simulink model "quadplane_sim_conf"  (R2023a)
settings: Solver=FixedStepAuto  StartTime=0.0  StopTime=100  FixedStep=0.001  RelTol=1e-9
undefined symbols (not defined in the file or in its folder): Aircraft, datetime, datevec, Earth, Env, Fmu, framePeriod_s, InitCond, Telem, WGS84
libraries: simulink x9, aerolibconvert2 x5, aerolibasang x3, aerolibtransform2 x2, aerolibatmos2 x1, aerolibgravity2 x1, sharedtransform x1, uavutilslib x1, aerolibadyn x1, fuzblock x1, shared6dof x1
(part 3 of 5)

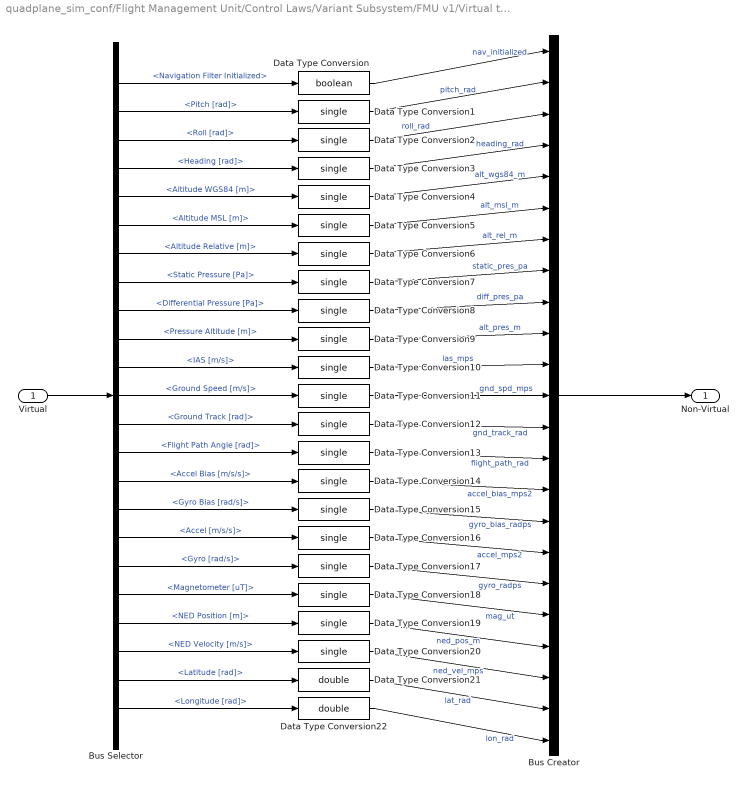
== system quadplane_sim_conf/Flight Management Unit/Control Laws/Variant Subsystem/FMU v1/Virtual to Non-Virtual Mapping2 ==
  Virtual : Inport
  Bus Creator : BusCreator  Inputs=23  OutDataTypeStr=Bus: NavData  NonVirtualBus=on
  Bus Selector : BusSelector  OutputSignals=Navigation Filter Initialized,Pitch [rad],Roll [rad],Heading [rad],Altitude WGS84 [m],Altitude MSL [m],Altitude Relative [m],Static Pressure [Pa],Differential Pressure [Pa],Pressure Altitude [m],IAS [m/s],Ground Speed [m/s],Ground Track [rad],Flight Path Angle [rad],Accel Bias [m/s/s],Gyro Bias [rad/s],Accel [m/s/s],Gyro [rad/s],Magnetometer [uT],NED Position [m],NED Velocity [m/s],Latitude [rad],Longitude [rad]
  Data Type Conversion : DataTypeConversion  OutDataTypeStr=boolean  SaturateOnIntegerOverflow=off  RndMeth=Floor
  Data Type Conversion{1..20} (20 alike) : DataTypeConversion  OutDataTypeStr=single  SaturateOnIntegerOverflow=off  RndMeth=Floor
  Data Type Conversion21 : DataTypeConversion  OutDataTypeStr=double  SaturateOnIntegerOverflow=off  RndMeth=Floor
  Data Type Conversion22 : DataTypeConversion  OutDataTypeStr=double  SaturateOnIntegerOverflow=off  RndMeth=Floor
  Non-Virtual : Outport  OutDataTypeStr=Bus: NavData
  wires:
  Data Type Conversion17/1 -> Bus Creator/18  "gyro_radps"
  Data Type Conversion22/1 -> Bus Creator/23  "lon_rad"
  Data Type Conversion21/1 -> Bus Creator/22  "lat_rad"
  Data Type Conversion20/1 -> Bus Creator/21  "ned_vel_mps"
  Data Type Conversion19/1 -> Bus Creator/20  "ned_pos_m"
  Data Type Conversion18/1 -> Bus Creator/19  "mag_ut"
  Data Type Conversion16/1 -> Bus Creator/17  "accel_mps2"
  Data Type Conversion15/1 -> Bus Creator/16  "gyro_bias_radps"
  Data Type Conversion14/1 -> Bus Creator/15  "accel_bias_mps2"
  Data Type Conversion13/1 -> Bus Creator/14  "flight_path_rad"
  Data Type Conversion12/1 -> Bus Creator/13  "gnd_track_rad"
  Data Type Conversion11/1 -> Bus Creator/12  "gnd_spd_mps"
  Data Type Conversion10/1 -> Bus Creator/11  "ias_mps"
  Data Type Conversion9/1 -> Bus Creator/10  "alt_pres_m"
  Data Type Conversion8/1 -> Bus Creator/9  "diff_pres_pa"
  Data Type Conversion7/1 -> Bus Creator/8  "static_pres_pa"
  Data Type Conversion6/1 -> Bus Creator/7  "alt_rel_m"
  Data Type Conversion5/1 -> Bus Creator/6  "alt_msl_m"
  Data Type Conversion4/1 -> Bus Creator/5  "alt_wgs84_m"
  Data Type Conversion3/1 -> Bus Creator/4  "heading_rad"
  Data Type Conversion2/1 -> Bus Creator/3  "roll_rad"
  Data Type Conversion1/1 -> Bus Creator/2  "pitch_rad"
  Data Type Conversion/1 -> Bus Creator/1  "nav_initialized"
  Bus Selector/23 -> Data Type Conversion22/1  "<Longitude [rad]>"
  Bus Selector/22 -> Data Type Conversion21/1  "<Latitude [rad]>"
  Bus Selector/21 -> Data Type Conversion20/1  "<NED Velocity [m/s]>"
  Bus Selector/20 -> Data Type Conversion19/1  "<NED Position [m]>"
  Bus Selector/19 -> Data Type Conversion18/1  "<Magnetometer [uT]>"
  Bus Selector/18 -> Data Type Conversion17/1  "<Gyro [rad/s]>"
  Bus Selector/17 -> Data Type Conversion16/1  "<Accel [m/s/s]>"
  Bus Selector/16 -> Data Type Conversion15/1  "<Gyro Bias [rad/s]>"
  Bus Selector/15 -> Data Type Conversion14/1  "<Accel Bias [m/s/s]>"
  Bus Selector/14 -> Data Type Conversion13/1  "<Flight Path Angle [rad]>"
  Bus Selector/13 -> Data Type Conversion12/1  "<Ground Track [rad]>"
  Bus Selector/12 -> Data Type Conversion11/1  "<Ground Speed [m/s]>"
  Bus Selector/11 -> Data Type Conversion10/1  "<IAS [m/s]>"
  Bus Selector/10 -> Data Type Conversion9/1  "<Pressure Altitude [m]>"
  Bus Selector/9 -> Data Type Conversion8/1  "<Differential Pressure [Pa]>"
  Bus Selector/8 -> Data Type Conversion7/1  "<Static Pressure [Pa]>"
  Bus Selector/7 -> Data Type Conversion6/1  "<Altitude Relative [m]>"
  Bus Selector/6 -> Data Type Conversion5/1  "<Altitude MSL [m]>"
  Bus Selector/5 -> Data Type Conversion4/1  "<Altitude WGS84 [m]>"
  Bus Selector/4 -> Data Type Conversion3/1  "<Heading [rad]>"
  Bus Selector/3 -> Data Type Conversion2/1  "<Roll [rad]>"
  Bus Selector/2 -> Data Type Conversion1/1  "<Pitch [rad]>"
  Bus Selector/1 -> Data Type Conversion/1  "<Navigation Filter Initialized>"
  Bus Creator/1 -> Non-Virtual/1
  Virtual/1 -> Bus Selector/1

== system quadplane_sim_conf/Flight Management Unit/Control Laws/Variant Subsystem/FMU v1/Virtual to Non-Virtual Mapping3 ==
  Virtual : Inport
  Bus Creator : BusCreator  Inputs=11  OutDataTypeStr=Bus: TelemData  NonVirtualBus=on
  Bus Selector : BusSelector  OutputSignals=Waypoints Updated,Fence Updated,Rally Points Updated,Current Waypoint Index,Number of Waypoints,Number of Fence Points,Number of Rally Points,Parameters,Flight Plan,Fence,Rally
  Data Type Conversion : DataTypeConversion  OutDataTypeStr=boolean  SaturateOnIntegerOverflow=off  RndMeth=Floor
  Data Type Conversion1 : DataTypeConversion  OutDataTypeStr=boolean  SaturateOnIntegerOverflow=off  RndMeth=Floor
  Data Type Conversion2 : DataTypeConversion  OutDataTypeStr=boolean  SaturateOnIntegerOverflow=off  RndMeth=Floor
  Data Type Conversion{3..6} (4 alike) : DataTypeConversion  OutDataTypeStr=int16  SaturateOnIntegerOverflow=off  RndMeth=Floor
  Data Type Conversion7 : DataTypeConversion  OutDataTypeStr=single  SaturateOnIntegerOverflow=off  RndMeth=Floor
  Signal Conversion : SignalConversion  ConversionOutput=Nonvirtual bus  OverrideOpt=off
  Signal Conversion1 : SignalConversion  ConversionOutput=Nonvirtual bus  OverrideOpt=off
  Signal Conversion2 : SignalConversion  ConversionOutput=Nonvirtual bus  OverrideOpt=off
  Non-Virtual : Outport  OutDataTypeStr=Bus: TelemData
  wires:
  Signal Conversion2/1 -> Bus Creator/11  "rally"
  Signal Conversion1/1 -> Bus Creator/10  "fence"
  Signal Conversion/1 -> Bus Creator/9  "flight_plan"
  Bus Selector/11 -> Signal Conversion2/1  "<Rally>"
  Bus Selector/10 -> Signal Conversion1/1  "<Fence>"
  Bus Selector/9 -> Signal Conversion/1  "<Flight Plan>"
  Data Type Conversion7/1 -> Bus Creator/8  "param"
  Data Type Conversion6/1 -> Bus Creator/7  "num_rally_points"
  Data Type Conversion5/1 -> Bus Creator/6  "num_fence_items"
  Data Type Conversion4/1 -> Bus Creator/5  "num_waypoints"
  Data Type Conversion3/1 -> Bus Creator/4  "current_waypoint"
  Data Type Conversion2/1 -> Bus Creator/3  "rally_points_updated"
  Data Type Conversion1/1 -> Bus Creator/2  "fence_updated"
  Data Type Conversion/1 -> Bus Creator/1  "waypoints_updated"
  Bus Selector/8 -> Data Type Conversion7/1  "<Parameters>"
  Bus Selector/7 -> Data Type Conversion6/1  "<Number of Rally Points>"
  Bus Selector/6 -> Data Type Conversion5/1  "<Number of Fence Points>"
  Bus Selector/5 -> Data Type Conversion4/1  "<Number of Waypoints>"
  Bus Selector/4 -> Data Type Conversion3/1  "<Current Waypoint Index>"
  Bus Selector/3 -> Data Type Conversion2/1  "<Rally Points Updated>"
  Bus Selector/2 -> Data Type Conversion1/1  "<Fence Updated>"
  Bus Selector/1 -> Data Type Conversion/1  "<Waypoints Updated>"
  Bus Creator/1 -> Non-Virtual/1
  Virtual/1 -> Bus Selector/1

== system quadplane_sim_conf/Flight Management Unit/Control Laws/Variant Subsystem/FMU v1/Virtual to Non-Virtual Mapping4 ==
  Non-Virtual : Inport  OutDataTypeStr=Bus: ControlData
  Bus Creator : BusCreator  Inputs=5
  Bus Selector : BusSelector  OutputSignals=waypoint_reached,mode,sbus,pwm,aux
  Data Type Conversion{1..4,22} (5 alike) : DataTypeConversion  OutDataTypeStr=double  SaturateOnIntegerOverflow=off  RndMeth=Floor
  Virtual : Outport
  wires:
  Data Type Conversion4/1 -> Bus Creator/5  "AUX"
  Data Type Conversion3/1 -> Bus Creator/4  "PWM"
  Bus Selector/5 -> Data Type Conversion4/1  "<aux>"
  Bus Selector/4 -> Data Type Conversion3/1  "<pwm>"
  Data Type Conversion2/1 -> Bus Creator/3  "SBUS"
  Bus Selector/3 -> Data Type Conversion2/1  "<sbus>"
  Data Type Conversion1/1 -> Bus Creator/2  "Mode"
  Bus Selector/2 -> Data Type Conversion1/1  "<mode>"
  Data Type Conversion22/1 -> Bus Creator/1  "Waypoint Reached"
  Bus Selector/1 -> Data Type Conversion22/1  "<waypoint_reached>"
  Bus Creator/1 -> Virtual/1
  Non-Virtual/1 -> Bus Selector/1

== system quadplane_sim_conf/Flight Management Unit/Control Laws/Variant Subsystem/FMU v1/Virtual to Non-Virtual Mapping5 ==
  Virtual : Inport
  Bus Creator : BusCreator  Inputs=7  OutDataTypeStr=Bus: SensorData  NonVirtualBus=on
  Bus Selector : BusSelector  OutputSignals=Pitot Static Installed,Inceptor,IMU,GNSS,Static Pressure,Differential Pressure,Analog
  Data Type Conversion : DataTypeConversion  OutDataTypeStr=boolean  SaturateOnIntegerOverflow=off  RndMeth=Floor
  Virtual to Non-Virtual Mapping1 : Subsystem
  Virtual to Non-Virtual Mapping2 : Subsystem
  Virtual to Non-Virtual Mapping3 : Subsystem
  Virtual to Non-Virtual Mapping4 : Subsystem
  Virtual to Non-Virtual Mapping5 : Subsystem
  Virtual to Non-Virtual Mapping6 : Subsystem
  Non-Virtual : Outport  OutDataTypeStr=Bus: SensorData
  wires:
  Virtual/1 -> Bus Selector/1
  Bus Creator/1 -> Non-Virtual/1
  Bus Selector/1 -> Data Type Conversion/1  "<Pitot Static Installed>"
  Data Type Conversion/1 -> Bus Creator/1  "pitot_static_installed"
  Bus Selector/2 -> Virtual to Non-Virtual Mapping1/1(Virtual)  "<Inceptor>"
  Virtual to Non-Virtual Mapping1/1(Non-Virtual) -> Bus Creator/2  "inceptor"
  Virtual to Non-Virtual Mapping2/1(Non-Virtual) -> Bus Creator/3  "imu"
  Bus Selector/3 -> Virtual to Non-Virtual Mapping2/1(Virtual)  "<IMU>"
  Virtual to Non-Virtual Mapping3/1(Non-Virtual) -> Bus Creator/4  "gnss"
  Bus Selector/4 -> Virtual to Non-Virtual Mapping3/1(Virtual)  "<GNSS>"
  Virtual to Non-Virtual Mapping4/1(Non-Virtual) -> Bus Creator/5  "static_pres"
  Bus Selector/5 -> Virtual to Non-Virtual Mapping4/1(Virtual)  "<Static Pressure>"
  Virtual to Non-Virtual Mapping5/1(Non-Virtual) -> Bus Creator/6  "diff_pres"
  Bus Selector/6 -> Virtual to Non-Virtual Mapping5/1(Virtual)  "<Differential Pressure>"
  Bus Selector/7 -> Virtual to Non-Virtual Mapping6/1(Virtual)  "<Analog>"
  Virtual to Non-Virtual Mapping6/1(Non-Virtual) -> Bus Creator/7  "adc"

== system quadplane_sim_conf/Flight Management Unit/Control Laws/Variant Subsystem/FMU v2/Virtual to Non-Virtual Mapping ==
  Virtual : Inport
  Bus Creator : BusCreator  Inputs=2  OutDataTypeStr=Bus: SysData  NonVirtualBus=on
  Bus Selector : BusSelector  OutputSignals=Frame Time [us],System Time [us]
  Data Type Conversion : DataTypeConversion  OutDataTypeStr=int32  SaturateOnIntegerOverflow=off  RndMeth=Floor
  Data Type Conversion5 : DataTypeConversion  OutDataTypeStr=int64  SaturateOnIntegerOverflow=off  RndMeth=Floor
  Non-Virtual : Outport  OutDataTypeStr=Bus: SysData
  wires:
  Bus Creator/1 -> Non-Virtual/1
  Virtual/1 -> Bus Selector/1
  Bus Selector/1 -> Data Type Conversion/1  "<Frame Time [us]>"
  Data Type Conversion/1 -> Bus Creator/1  "frame_time_us"
  Bus Selector/2 -> Data Type Conversion5/1  "<System Time [us]>"
  Data Type Conversion5/1 -> Bus Creator/2  "sys_time_us"

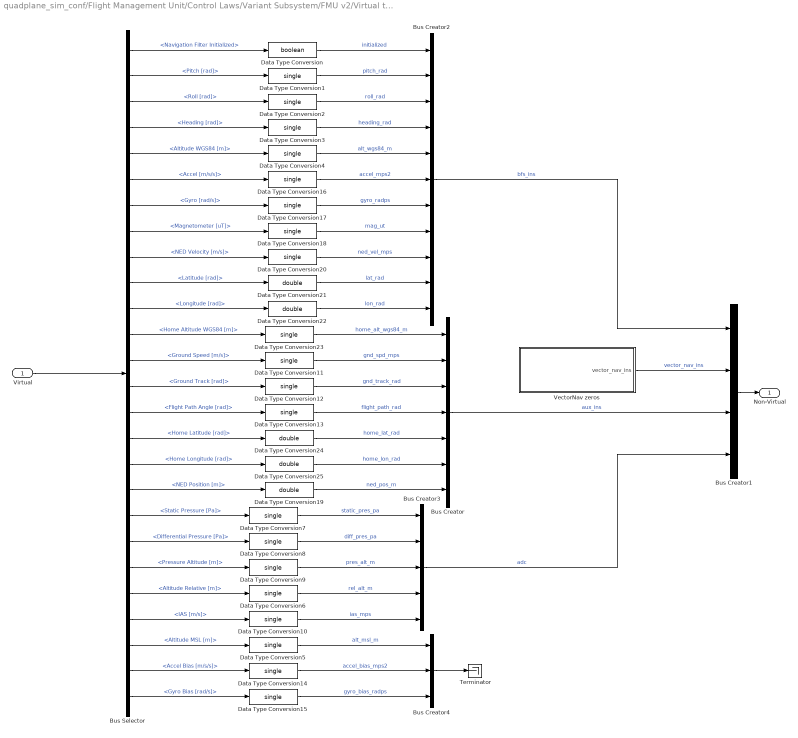
== system quadplane_sim_conf/Flight Management Unit/Control Laws/Variant Subsystem/FMU v2/Virtual to Non-Virtual Mapping1 ==
  Virtual : Inport
  Bus Creator : BusCreator  Inputs=7  OutDataTypeStr=Bus: AuxInsData
  Bus Creator1 : BusCreator  Inputs=4  OutDataTypeStr=Bus: StateEstData
  Bus Creator2 : BusCreator  Inputs=11  OutDataTypeStr=Bus: InsData
  Bus Creator3 : BusCreator  Inputs=5  OutDataTypeStr=Bus: AdcData
  Bus Creator4 : BusCreator  Inputs=3
  Bus Selector : BusSelector  OutputSignals=Navigation Filter Initialized,Pitch [rad],Roll [rad],Heading [rad],Altitude WGS84 [m],Accel [m/s/s],Gyro [rad/s],Magnetometer [uT],NED Velocity [m/s],Latitude [rad],Longitude [rad],Home Altitude WGS84 [m],Ground Speed [m/s],Ground Track [rad],Flight Path Angle [rad],Home Latitude [rad],Home Longitude [rad],NED Position [m],Static Pressure [Pa],Differential Pressure [Pa],Pressure Altitude [m],Altitude Relative [m],IAS [m/s],Altitude MSL [m],Accel Bias [m/s/s],Gyro Bias [rad/s]
  Data Type Conversion : DataTypeConversion  OutDataTypeStr=boolean  SaturateOnIntegerOverflow=off  RndMeth=Floor
  Data Type Conversion{1..18,20,23} (20 alike) : DataTypeConversion  OutDataTypeStr=single  SaturateOnIntegerOverflow=off  RndMeth=Floor
  Data Type Conversion{19,21..22,24..25} (5 alike) : DataTypeConversion  OutDataTypeStr=double  SaturateOnIntegerOverflow=off  RndMeth=Floor
  Terminator : Terminator
  VectorNav zeros : Subsystem
  Non-Virtual : Outport  OutDataTypeStr=Bus: StateEstData
  wires:
  Virtual/1 -> Bus Selector/1
  Bus Selector/1 -> Data Type Conversion/1  "<Navigation Filter Initialized>"
  Bus Selector/2 -> Data Type Conversion1/1  "<Pitch [rad]>"
  Bus Selector/3 -> Data Type Conversion2/1  "<Roll [rad]>"
  Bus Selector/4 -> Data Type Conversion3/1  "<Heading [rad]>"
  Bus Selector/5 -> Data Type Conversion4/1  "<Altitude WGS84 [m]>"
  Bus Selector/24 -> Data Type Conversion5/1  "<Altitude MSL [m]>"
  Bus Selector/22 -> Data Type Conversion6/1  "<Altitude Relative [m]>"
  Bus Selector/19 -> Data Type Conversion7/1  "<Static Pressure [Pa]>"
  Bus Selector/20 -> Data Type Conversion8/1  "<Differential Pressure [Pa]>"
  Bus Selector/21 -> Data Type Conversion9/1  "<Pressure Altitude [m]>"
  Bus Selector/23 -> Data Type Conversion10/1  "<IAS [m/s]>"
  Bus Selector/13 -> Data Type Conversion11/1  "<Ground Speed [m/s]>"
  Bus Selector/14 -> Data Type Conversion12/1  "<Ground Track [rad]>"
  Bus Selector/15 -> Data Type Conversion13/1  "<Flight Path Angle [rad]>"
  Bus Selector/25 -> Data Type Conversion14/1  "<Accel Bias [m/s/s]>"
  Bus Selector/26 -> Data Type Conversion15/1  "<Gyro Bias [rad/s]>"
  Bus Selector/6 -> Data Type Conversion16/1  "<Accel [m/s/s]>"
  Bus Selector/7 -> Data Type Conversion17/1  "<Gyro [rad/s]>"
  Bus Selector/8 -> Data Type Conversion18/1  "<Magnetometer [uT]>"
  Bus Selector/18 -> Data Type Conversion19/1  "<NED Position [m]>"
  Bus Selector/9 -> Data Type Conversion20/1  "<NED Velocity [m/s]>"
  Bus Selector/10 -> Data Type Conversion21/1  "<Latitude [rad]>"
  Bus Selector/11 -> Data Type Conversion22/1  "<Longitude [rad]>"
  Data Type Conversion/1 -> Bus Creator2/1  "initialized"
  Data Type Conversion1/1 -> Bus Creator2/2  "pitch_rad"
  Data Type Conversion2/1 -> Bus Creator2/3  "roll_rad"
  Data Type Conversion3/1 -> Bus Creator2/4  "heading_rad"
  Data Type Conversion4/1 -> Bus Creator2/5  "alt_wgs84_m"
  Data Type Conversion22/1 -> Bus Creator2/11  "lon_rad"
  Data Type Conversion21/1 -> Bus Creator2/10  "lat_rad"
  Data Type Conversion20/1 -> Bus Creator2/9  "ned_vel_mps"
  Data Type Conversion19/1 -> Bus Creator/7  "ned_pos_m"
  Data Type Conversion18/1 -> Bus Creator2/8  "mag_ut"
  Data Type Conversion17/1 -> Bus Creator2/7  "gyro_radps"
  Data Type Conversion16/1 -> Bus Creator2/6  "accel_mps2"
  Data Type Conversion15/1 -> Bus Creator4/3  "gyro_bias_radps"
  Data Type Conversion14/1 -> Bus Creator4/2  "accel_bias_mps2"
  Data Type Conversion13/1 -> Bus Creator/4  "flight_path_rad"
  Data Type Conversion12/1 -> Bus Creator/3  "gnd_track_rad"
  Data Type Conversion11/1 -> Bus Creator/2  "gnd_spd_mps"
  Data Type Conversion10/1 -> Bus Creator3/5  "ias_mps"
  Data Type Conversion9/1 -> Bus Creator3/3  "pres_alt_m"
  Data Type Conversion8/1 -> Bus Creator3/2  "diff_pres_pa"
  Data Type Conversion7/1 -> Bus Creator3/1  "static_pres_pa"
  Data Type Conversion6/1 -> Bus Creator3/4  "rel_alt_m"
  Bus Selector/12 -> Data Type Conversion23/1  "<Home Altitude WGS84 [m]>"
  Data Type Conversion23/1 -> Bus Creator/1  "home_alt_wgs84_m"
  Bus Selector/16 -> Data Type Conversion24/1  "<Home Latitude [rad]>"
  Bus Selector/17 -> Data Type Conversion25/1  "<Home Longitude [rad]>"
  Data Type Conversion24/1 -> Bus Creator/5  "home_lat_rad"
  Data Type Conversion25/1 -> Bus Creator/6  "home_lon_rad"
  Bus Creator1/1 -> Non-Virtual/1
  Bus Creator2/1 -> Bus Creator1/1  "bfs_ins"
  Data Type Conversion5/1 -> Bus Creator4/1  "alt_msl_m"
  Bus Creator/1 -> Bus Creator1/3  "aux_ins"
  Bus Creator3/1 -> Bus Creator1/4  "adc"
  Bus Creator4/1 -> Terminator/1
  VectorNav zeros/1(vector_nav_ins) -> Bus Creator1/2  "vector_nav_ins"

== system quadplane_sim_conf/Flight Management Unit/Control Laws/Variant Subsystem/FMU v2/Virtual to Non-Virtual Mapping3 ==
  Virtual : Inport
  Bus Creator : BusCreator  Inputs=11  OutDataTypeStr=Bus: TelemData  NonVirtualBus=on
  Bus Selector : BusSelector  OutputSignals=Waypoints Updated,Fence Updated,Rally Points Updated,Current Waypoint Index,Number of Waypoints,Number of Fence Points,Number of Rally Points,Parameters,Flight Plan,Fence,Rally
  Data Type Conversion : DataTypeConversion  OutDataTypeStr=boolean  SaturateOnIntegerOverflow=off  RndMeth=Floor
  Data Type Conversion1 : DataTypeConversion  OutDataTypeStr=boolean  SaturateOnIntegerOverflow=off  RndMeth=Floor
  Data Type Conversion2 : DataTypeConversion  OutDataTypeStr=boolean  SaturateOnIntegerOverflow=off  RndMeth=Floor
  Data Type Conversion{3..6} (4 alike) : DataTypeConversion  OutDataTypeStr=int16  SaturateOnIntegerOverflow=off  RndMeth=Floor
  Data Type Conversion7 : DataTypeConversion  OutDataTypeStr=single  SaturateOnIntegerOverflow=off  RndMeth=Floor
  Signal Conversion : SignalConversion  ConversionOutput=Nonvirtual bus  OutDataTypeStr=Bus: MissionItem  OverrideOpt=off
  Signal Conversion1 : SignalConversion  ConversionOutput=Nonvirtual bus  OutDataTypeStr=Bus: MissionItem  OverrideOpt=off
  Signal Conversion2 : SignalConversion  ConversionOutput=Nonvirtual bus  OutDataTypeStr=Bus: MissionItem  OverrideOpt=off
  Non-Virtual : Outport  OutDataTypeStr=Bus: TelemData
  wires:
  Virtual/1 -> Bus Selector/1
  Bus Creator/1 -> Non-Virtual/1
  Bus Selector/1 -> Data Type Conversion/1  "<Waypoints Updated>"
  Bus Selector/2 -> Data Type Conversion1/1  "<Fence Updated>"
  Bus Selector/3 -> Data Type Conversion2/1  "<Rally Points Updated>"
  Bus Selector/4 -> Data Type Conversion3/1  "<Current Waypoint Index>"
  Bus Selector/5 -> Data Type Conversion4/1  "<Number of Waypoints>"
  Bus Selector/6 -> Data Type Conversion5/1  "<Number of Fence Points>"
  Bus Selector/7 -> Data Type Conversion6/1  "<Number of Rally Points>"
  Bus Selector/8 -> Data Type Conversion7/1  "<Parameters>"
  Data Type Conversion/1 -> Bus Creator/1  "waypoints_updated"
  Data Type Conversion1/1 -> Bus Creator/2  "fence_updated"
  Data Type Conversion2/1 -> Bus Creator/3  "rally_points_updated"
  Data Type Conversion3/1 -> Bus Creator/4  "current_waypoint"
  Data Type Conversion4/1 -> Bus Creator/5  "num_waypoints"
  Data Type Conversion5/1 -> Bus Creator/6  "num_fence_items"
  Data Type Conversion6/1 -> Bus Creator/7  "num_rally_points"
  Data Type Conversion7/1 -> Bus Creator/8  "param"
  Bus Selector/9 -> Signal Conversion/1  "<Flight Plan>"
  Bus Selector/10 -> Signal Conversion1/1  "<Fence>"
  Bus Selector/11 -> Signal Conversion2/1  "<Rally>"
  Signal Conversion/1 -> Bus Creator/9  "flight_plan"
  Signal Conversion1/1 -> Bus Creator/10  "fence"
  Signal Conversion2/1 -> Bus Creator/11  "rally"

== system quadplane_sim_conf/Flight Management Unit/Control Laws/Variant Subsystem/FMU v2/Virtual to Non-Virtual Mapping4 ==
  Non-Virtual1 : Inport  OutDataTypeStr=Bus: VmsData
  Bus Creator1 : BusCreator  Inputs=9
  Bus Selector1 : BusSelector  OutputSignals=advance_waypoint,motors_enabled,mode,sbus,pwm,throttle_cmd_prcnt,flight_time_remaining_s,power_remaining_prcnt,aux
  Cast To Boolean : DataTypeConversion  OutDataTypeStr=boolean  SaturateOnIntegerOverflow=off  RndMeth=Floor
  Cast To Boolean1 : DataTypeConversion  OutDataTypeStr=boolean  SaturateOnIntegerOverflow=off  RndMeth=Floor
  Cast To Boolean2 : DataTypeConversion  OutDataTypeStr=int8  SaturateOnIntegerOverflow=off  RndMeth=Floor
  Cast To Boolean3 : DataTypeConversion  OutDataTypeStr=int16  SaturateOnIntegerOverflow=off  RndMeth=Floor
  Cast To Boolean4 : DataTypeConversion  OutDataTypeStr=int16  SaturateOnIntegerOverflow=off  RndMeth=Floor
  Cast To Boolean{5..8} (4 alike) : DataTypeConversion  OutDataTypeStr=single  SaturateOnIntegerOverflow=off  RndMeth=Floor
  Virtual1 : Outport
  wires:
  Non-Virtual1/1 -> Bus Selector1/1
  Bus Creator1/1 -> Virtual1/1
  Bus Selector1/1 -> Cast To Boolean/1  "<advance_waypoint>"
  Bus Selector1/2 -> Cast To Boolean1/1  "<motors_enabled>"
  Bus Selector1/3 -> Cast To Boolean2/1  "<mode>"
  Bus Selector1/4 -> Cast To Boolean3/1  "<sbus>"
  Bus Selector1/5 -> Cast To Boolean4/1  "<pwm>"
  Bus Selector1/6 -> Cast To Boolean5/1  "<throttle_cmd_prcnt>"
  Bus Selector1/7 -> Cast To Boolean6/1  "<flight_time_remaining_s>"
  Bus Selector1/8 -> Cast To Boolean7/1  "<power_remaining_prcnt>"
  Bus Selector1/9 -> Cast To Boolean8/1  "<aux>"
  Cast To Boolean/1 -> Bus Creator1/1  "advance_waypoint"
  Cast To Boolean1/1 -> Bus Creator1/2  "motors-enabled"
  Cast To Boolean2/1 -> Bus Creator1/3  "mode"
  Cast To Boolean3/1 -> Bus Creator1/4  "sbus"
  Cast To Boolean4/1 -> Bus Creator1/5  "pwm"
  Cast To Boolean5/1 -> Bus Creator1/6  "throttle_cmd_prcnt"
  Cast To Boolean6/1 -> Bus Creator1/7  "flight_time_remaining_s"
  Cast To Boolean7/1 -> Bus Creator1/8  "power_remaining_prcnt"
  Cast To Boolean8/1 -> Bus Creator1/9  "aux"

== system quadplane_sim_conf/Flight Management Unit/Control Laws/Variant Subsystem/FMU v2/Virtual to Non-Virtual Mapping5 ==
  Virtual : Inport
  Bus Creator : BusCreator  Inputs=18  OutDataTypeStr=Bus: SensorData
  Bus Selector : BusSelector  OutputSignals=Pitot Static Installed,Inceptor,IMU,Static Pressure,GNSS,Differential Pressure,Analog,Battery
  Subsystem : Subsystem
  Subsystem1 : Subsystem
  Subsystem2 : Subsystem
  Subsystem3 : Subsystem
  Subsystem4 : Subsystem
  Subsystem5 : Subsystem
  Subsystem6 : Subsystem
  Subsystem7 : Subsystem
  ZEROS : Subsystem
  Non-Virtual : Outport  OutDataTypeStr=Bus: SensorData
  wires:
  Virtual/1 -> Bus Selector/1
  Bus Creator/1 -> Non-Virtual/1
  Bus Selector/1 -> [pitot_static_installed]  "<Pitot Static Installed>"
  Bus Selector/2 -> Subsystem/1(In1)  "<Inceptor>"
  Subsystem/1(Out1) -> Bus Creator/1
  Bus Selector/7 -> Subsystem1/1(In1)  "<Analog>"
  Bus Selector/3 -> Subsystem6/1(In1), Subsystem5/1(In1)  "<IMU>"
  Bus Selector/5 -> Subsystem7/1(In1)  "<GNSS>"
  Subsystem1/1(Out1) -> Bus Creator/17
  Bus Selector/8 -> Subsystem2/1(<Battery>)  "<Battery>"
  Subsystem2/1(Out1) -> Bus Creator/18
  Bus Selector/4 -> Subsystem3/1(In1)  "<Static Pressure>"
  Bus Selector/6 -> Subsystem4/2(In1)  "<Differential Pressure>"
  Subsystem7/1(Out1) -> Bus Creator/10
  Subsystem4/1(Out1) -> Bus Creator/13
  Subsystem3/1(Out1) -> Bus Creator/4
  Subsystem5/1(Out1) -> Bus Creator/2
  Subsystem6/1(Out1) -> Bus Creator/3
  ZEROS/3(GNSS) -> Bus Creator/11, Bus Creator/8
  ZEROS/4(ExtPres) -> Bus Creator/7, Bus Creator/15, Bus Creator/14, Bus Creator/12
  ZEROS/2(MAG) -> Bus Creator/9, Bus Creator/6
  ZEROS/1(IMU) -> Bus Creator/5
  ZEROS/5(RadAlt) -> Bus Creator/16
  [pitot_static_installed] -> Subsystem4/1(In2)

== system quadplane_sim_conf/Flight Management Unit/Control Laws/Variant Subsystem/FMU v2 Beta/Virtual to Non-Virtual Mapping ==
  Virtual : Inport
  Bus Creator : BusCreator  Inputs=4  OutDataTypeStr=Bus: SysData  NonVirtualBus=on
  Bus Selector : BusSelector  OutputSignals=Frame Time [us],Frame Time [s],System Time [us],System Time [s]
  Data Type Conversion : DataTypeConversion  OutDataTypeStr=int32  SaturateOnIntegerOverflow=off  RndMeth=Floor
  Data Type Conversion5 : DataTypeConversion  OutDataTypeStr=int64  SaturateOnIntegerOverflow=off  RndMeth=Floor
  Data Type Conversion6 : DataTypeConversion  OutDataTypeStr=single  SaturateOnIntegerOverflow=off  RndMeth=Floor
  Data Type Conversion7 : DataTypeConversion  OutDataTypeStr=double  SaturateOnIntegerOverflow=off  RndMeth=Floor
  Non-Virtual : Outport  OutDataTypeStr=Bus: SysData
  wires:
  Bus Creator/1 -> Non-Virtual/1
  Virtual/1 -> Bus Selector/1
  Bus Selector/1 -> Data Type Conversion/1  "<Frame Time [us]>"
  Data Type Conversion/1 -> Bus Creator/1  "frame_time_us"
  Bus Selector/3 -> Data Type Conversion5/1  "<System Time [us]>"
  Data Type Conversion5/1 -> Bus Creator/3  "sys_time_us"
  Bus Selector/2 -> Data Type Conversion6/1  "<Frame Time [s]>"
  Data Type Conversion6/1 -> Bus Creator/2  "frame_time_s"
  Bus Selector/4 -> Data Type Conversion7/1  "<System Time [s]>"
  Data Type Conversion7/1 -> Bus Creator/4  "sys_time_s"

== system quadplane_sim_conf/Flight Management Unit/Control Laws/Variant Subsystem/FMU v2 Beta/Virtual to Non-Virtual Mapping1 ==
  Virtual : Inport
  Bus Creator : BusCreator  Inputs=7  OutDataTypeStr=Bus: SensorData  NonVirtualBus=on
  Bus Selector : BusSelector  OutputSignals=Pitot Static Installed,Inceptor,IMU,GNSS,Static Pressure,Differential Pressure,Analog
  Data Type Conversion : DataTypeConversion  OutDataTypeStr=boolean  SaturateOnIntegerOverflow=off  RndMeth=Floor
  Virtual to Non-Virtual Mapping1 : Subsystem
  Virtual to Non-Virtual Mapping2 : Subsystem
  Virtual to Non-Virtual Mapping3 : Subsystem
  Virtual to Non-Virtual Mapping4 : Subsystem
  Virtual to Non-Virtual Mapping5 : Subsystem
  Virtual to Non-Virtual Mapping6 : Subsystem
  Non-Virtual : Outport  OutDataTypeStr=Bus: SensorData
  wires:
  Virtual/1 -> Bus Selector/1
  Bus Creator/1 -> Non-Virtual/1
  Bus Selector/1 -> Data Type Conversion/1  "<Pitot Static Installed>"
  Data Type Conversion/1 -> Bus Creator/1  "pitot_static_installed"
  Bus Selector/2 -> Virtual to Non-Virtual Mapping1/1(Virtual)  "<Inceptor>"
  Virtual to Non-Virtual Mapping1/1(Non-Virtual) -> Bus Creator/2  "inceptor"
  Virtual to Non-Virtual Mapping2/1(Non-Virtual) -> Bus Creator/3  "imu"
  Bus Selector/3 -> Virtual to Non-Virtual Mapping2/1(Virtual)  "<IMU>"
  Virtual to Non-Virtual Mapping3/1(Non-Virtual) -> Bus Creator/4  "gnss"
  Bus Selector/4 -> Virtual to Non-Virtual Mapping3/1(Virtual)  "<GNSS>"
  Virtual to Non-Virtual Mapping4/1(Non-Virtual) -> Bus Creator/5  "static_pres"
  Bus Selector/5 -> Virtual to Non-Virtual Mapping4/1(Virtual)  "<Static Pressure>"
  Virtual to Non-Virtual Mapping5/1(Non-Virtual) -> Bus Creator/6  "diff_pres"
  Bus Selector/6 -> Virtual to Non-Virtual Mapping5/1(Virtual)  "<Differential Pressure>"
  Bus Selector/7 -> Virtual to Non-Virtual Mapping6/1(Virtual)  "<Analog>"
  Virtual to Non-Virtual Mapping6/1(Non-Virtual) -> Bus Creator/7  "analog"

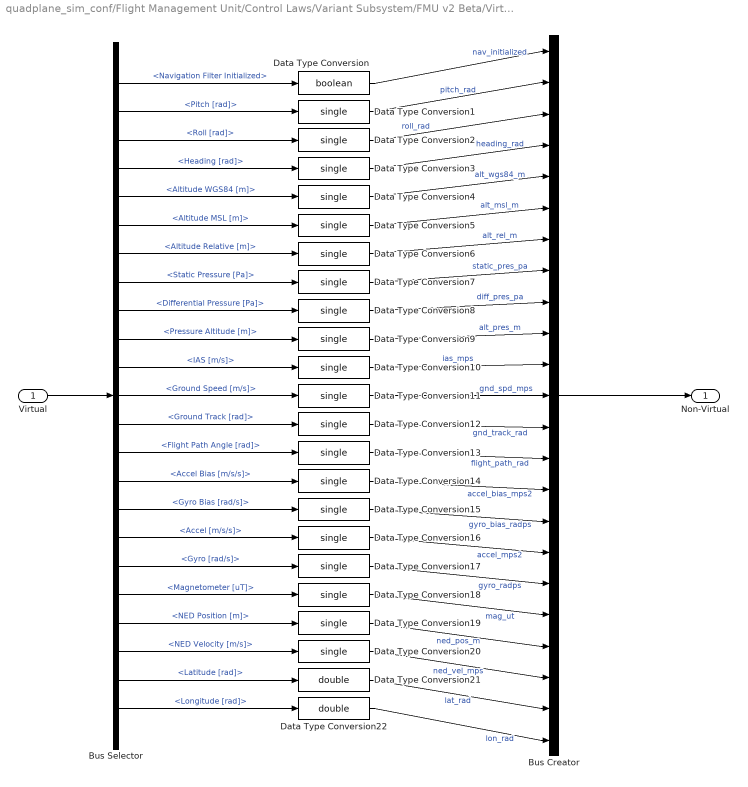
== system quadplane_sim_conf/Flight Management Unit/Control Laws/Variant Subsystem/FMU v2 Beta/Virtual to Non-Virtual Mapping2 ==
  Virtual : Inport
  Bus Creator : BusCreator  Inputs=23  OutDataTypeStr=Bus: NavData  NonVirtualBus=on
  Bus Selector : BusSelector  OutputSignals=Navigation Filter Initialized,Pitch [rad],Roll [rad],Heading [rad],Altitude WGS84 [m],Altitude MSL [m],Altitude Relative [m],Static Pressure [Pa],Differential Pressure [Pa],Pressure Altitude [m],IAS [m/s],Ground Speed [m/s],Ground Track [rad],Flight Path Angle [rad],Accel Bias [m/s/s],Gyro Bias [rad/s],Accel [m/s/s],Gyro [rad/s],Magnetometer [uT],NED Position [m],NED Velocity [m/s],Latitude [rad],Longitude [rad]
  Data Type Conversion : DataTypeConversion  OutDataTypeStr=boolean  SaturateOnIntegerOverflow=off  RndMeth=Floor
  Data Type Conversion{1..20} (20 alike) : DataTypeConversion  OutDataTypeStr=single  SaturateOnIntegerOverflow=off  RndMeth=Floor
  Data Type Conversion21 : DataTypeConversion  OutDataTypeStr=double  SaturateOnIntegerOverflow=off  RndMeth=Floor
  Data Type Conversion22 : DataTypeConversion  OutDataTypeStr=double  SaturateOnIntegerOverflow=off  RndMeth=Floor
  Non-Virtual : Outport  OutDataTypeStr=Bus: NavData
  wires:
  Virtual/1 -> Bus Selector/1
  Bus Creator/1 -> Non-Virtual/1
  Bus Selector/1 -> Data Type Conversion/1  "<Navigation Filter Initialized>"
  Bus Selector/2 -> Data Type Conversion1/1  "<Pitch [rad]>"
  Bus Selector/3 -> Data Type Conversion2/1  "<Roll [rad]>"
  Bus Selector/4 -> Data Type Conversion3/1  "<Heading [rad]>"
  Bus Selector/5 -> Data Type Conversion4/1  "<Altitude WGS84 [m]>"
  Bus Selector/6 -> Data Type Conversion5/1  "<Altitude MSL [m]>"
  Bus Selector/7 -> Data Type Conversion6/1  "<Altitude Relative [m]>"
  Bus Selector/8 -> Data Type Conversion7/1  "<Static Pressure [Pa]>"
  Bus Selector/9 -> Data Type Conversion8/1  "<Differential Pressure [Pa]>"
  Bus Selector/10 -> Data Type Conversion9/1  "<Pressure Altitude [m]>"
  Bus Selector/11 -> Data Type Conversion10/1  "<IAS [m/s]>"
  Bus Selector/12 -> Data Type Conversion11/1  "<Ground Speed [m/s]>"
  Bus Selector/13 -> Data Type Conversion12/1  "<Ground Track [rad]>"
  Bus Selector/14 -> Data Type Conversion13/1  "<Flight Path Angle [rad]>"
  Bus Selector/15 -> Data Type Conversion14/1  "<Accel Bias [m/s/s]>"
  Bus Selector/16 -> Data Type Conversion15/1  "<Gyro Bias [rad/s]>"
  Bus Selector/17 -> Data Type Conversion16/1  "<Accel [m/s/s]>"
  Bus Selector/18 -> Data Type Conversion17/1  "<Gyro [rad/s]>"
  Bus Selector/19 -> Data Type Conversion18/1  "<Magnetometer [uT]>"
  Bus Selector/20 -> Data Type Conversion19/1  "<NED Position [m]>"
  Bus Selector/21 -> Data Type Conversion20/1  "<NED Velocity [m/s]>"
  Bus Selector/22 -> Data Type Conversion21/1  "<Latitude [rad]>"
  Bus Selector/23 -> Data Type Conversion22/1  "<Longitude [rad]>"
  Data Type Conversion/1 -> Bus Creator/1  "nav_initialized"
  Data Type Conversion1/1 -> Bus Creator/2  "pitch_rad"
  Data Type Conversion2/1 -> Bus Creator/3  "roll_rad"
  Data Type Conversion3/1 -> Bus Creator/4  "heading_rad"
  Data Type Conversion4/1 -> Bus Creator/5  "alt_wgs84_m"
  Data Type Conversion5/1 -> Bus Creator/6  "alt_msl_m"
  Data Type Conversion6/1 -> Bus Creator/7  "alt_rel_m"
  Data Type Conversion7/1 -> Bus Creator/8  "static_pres_pa"
  Data Type Conversion8/1 -> Bus Creator/9  "diff_pres_pa"
  Data Type Conversion9/1 -> Bus Creator/10  "alt_pres_m"
  Data Type Conversion10/1 -> Bus Creator/11  "ias_mps"
  Data Type Conversion11/1 -> Bus Creator/12  "gnd_spd_mps"
  Data Type Conversion12/1 -> Bus Creator/13  "gnd_track_rad"
  Data Type Conversion13/1 -> Bus Creator/14  "flight_path_rad"
  Data Type Conversion14/1 -> Bus Creator/15  "accel_bias_mps2"
  Data Type Conversion15/1 -> Bus Creator/16  "gyro_bias_radps"
  Data Type Conversion16/1 -> Bus Creator/17  "accel_mps2"
  Data Type Conversion18/1 -> Bus Creator/19  "mag_ut"
  Data Type Conversion19/1 -> Bus Creator/20  "ned_pos_m"
  Data Type Conversion20/1 -> Bus Creator/21  "ned_vel_mps"
  Data Type Conversion21/1 -> Bus Creator/22  "lat_rad"
  Data Type Conversion22/1 -> Bus Creator/23  "lon_rad"
  Data Type Conversion17/1 -> Bus Creator/18  "gyro_radps"

== system quadplane_sim_conf/Flight Management Unit/Control Laws/Variant Subsystem/FMU v2 Beta/Virtual to Non-Virtual Mapping3 ==
  Virtual : Inport
  Bus Creator : BusCreator  Inputs=11  OutDataTypeStr=Bus: TelemData  NonVirtualBus=on
  Bus Selector : BusSelector  OutputSignals=Waypoints Updated,Fence Updated,Rally Points Updated,Current Waypoint Index,Number of Waypoints,Number of Fence Points,Number of Rally Points,Parameters,Flight Plan,Fence,Rally
  Data Type Conversion : DataTypeConversion  OutDataTypeStr=boolean  SaturateOnIntegerOverflow=off  RndMeth=Floor
  Data Type Conversion1 : DataTypeConversion  OutDataTypeStr=boolean  SaturateOnIntegerOverflow=off  RndMeth=Floor
  Data Type Conversion2 : DataTypeConversion  OutDataTypeStr=boolean  SaturateOnIntegerOverflow=off  RndMeth=Floor
  Data Type Conversion{3..6} (4 alike) : DataTypeConversion  OutDataTypeStr=int16  SaturateOnIntegerOverflow=off  RndMeth=Floor
  Data Type Conversion7 : DataTypeConversion  OutDataTypeStr=single  SaturateOnIntegerOverflow=off  RndMeth=Floor
  Signal Conversion : SignalConversion  ConversionOutput=Nonvirtual bus  OverrideOpt=off
  Signal Conversion1 : SignalConversion  ConversionOutput=Nonvirtual bus  OverrideOpt=off
  Signal Conversion2 : SignalConversion  ConversionOutput=Nonvirtual bus  OverrideOpt=off
  Non-Virtual : Outport  OutDataTypeStr=Bus: TelemData
  wires:
  Virtual/1 -> Bus Selector/1
  Bus Creator/1 -> Non-Virtual/1
  Bus Selector/1 -> Data Type Conversion/1  "<Waypoints Updated>"
  Bus Selector/2 -> Data Type Conversion1/1  "<Fence Updated>"
  Bus Selector/3 -> Data Type Conversion2/1  "<Rally Points Updated>"
  Bus Selector/4 -> Data Type Conversion3/1  "<Current Waypoint Index>"
  Bus Selector/5 -> Data Type Conversion4/1  "<Number of Waypoints>"
  Bus Selector/6 -> Data Type Conversion5/1  "<Number of Fence Points>"
  Bus Selector/7 -> Data Type Conversion6/1  "<Number of Rally Points>"
  Bus Selector/8 -> Data Type Conversion7/1  "<Parameters>"
  Data Type Conversion/1 -> Bus Creator/1  "waypoints_updated"
  Data Type Conversion1/1 -> Bus Creator/2  "fence_updated"
  Data Type Conversion2/1 -> Bus Creator/3  "rally_points_updated"
  Data Type Conversion3/1 -> Bus Creator/4  "current_waypoint"
  Data Type Conversion4/1 -> Bus Creator/5  "num_waypoints"
  Data Type Conversion5/1 -> Bus Creator/6  "num_fence_items"
  Data Type Conversion6/1 -> Bus Creator/7  "num_rally_points"
  Data Type Conversion7/1 -> Bus Creator/8  "param"
  Bus Selector/9 -> Signal Conversion/1  "<Flight Plan>"
  Bus Selector/10 -> Signal Conversion1/1  "<Fence>"
  Bus Selector/11 -> Signal Conversion2/1  "<Rally>"
  Signal Conversion/1 -> Bus Creator/9  "flight_plan"
  Signal Conversion1/1 -> Bus Creator/10  "fence"
  Signal Conversion2/1 -> Bus Creator/11  "rally"

== system quadplane_sim_conf/Flight Management Unit/Control Laws/Variant Subsystem/FMU v2 Beta/Virtual to Non-Virtual Mapping4 ==
  Non-Virtual : Inport  OutDataTypeStr=Bus: ControlData
  Bus Creator : BusCreator  Inputs=5
  Bus Selector : BusSelector  OutputSignals=waypoint_reached,mode,sbus,pwm,aux
  Data Type Conversion{1..4,22} (5 alike) : DataTypeConversion  OutDataTypeStr=double  SaturateOnIntegerOverflow=off  RndMeth=Floor
  Virtual : Outport
  wires:
  Non-Virtual/1 -> Bus Selector/1
  Bus Creator/1 -> Virtual/1
  Bus Selector/1 -> Data Type Conversion22/1  "<waypoint_reached>"
  Data Type Conversion22/1 -> Bus Creator/1  "Waypoint Reached"
  Bus Selector/2 -> Data Type Conversion1/1  "<mode>"
  Data Type Conversion1/1 -> Bus Creator/2  "Mode"
  Bus Selector/3 -> Data Type Conversion2/1  "<sbus>"
  Data Type Conversion2/1 -> Bus Creator/3  "SBUS"
  Bus Selector/4 -> Data Type Conversion3/1  "<pwm>"
  Bus Selector/5 -> Data Type Conversion4/1  "<aux>"
  Data Type Conversion3/1 -> Bus Creator/4  "PWM"
  Data Type Conversion4/1 -> Bus Creator/5  "AUX"

== system quadplane_sim_conf/Flight Management Unit/Sensor Models/GNSS/Triggered Subsystem/Norm ==
  2D Vector : Inport
  Product : Product
  Sqrt : Sqrt
  Sum of Elements : Sum  Inputs=+
  Norm : Outport
  wires:
  2D Vector/1 -> Product/2, Product/1
  Product/1 -> Sum of Elements/1
  Sum of Elements/1 -> Sqrt/1
  Sqrt/1 -> Norm/1

== system quadplane_sim_conf/Flight Management Unit/Control Laws/Variant Subsystem/FMU Mini/Virtual to Non-Virtual Mapping4/Subsystem1 ==
  Non-Virtual : Inport  OutDataTypeStr=Bus: BatteryData
  Bus Creator : BusCreator  Inputs=5
  Bus Selector : BusSelector  OutputSignals=voltage_v,current_ma,consumed_mah,remaining_prcnt,remaining_time_s
  Data Type Conversion{,1..4} (5 alike) : DataTypeConversion  OutDataTypeStr=double  SaturateOnIntegerOverflow=off  RndMeth=Floor
  Virtual : Outport
  wires:
  Non-Virtual/1 -> Bus Selector/1
  Bus Selector/1 -> Data Type Conversion/1  "<voltage_v>"
  Bus Selector/2 -> Data Type Conversion1/1  "<current_ma>"
  Bus Selector/3 -> Data Type Conversion2/1  "<consumed_mah>"
  Bus Selector/4 -> Data Type Conversion3/1  "<remaining_prcnt>"
  Bus Selector/5 -> Data Type Conversion4/1  "<remaining_time_s>"
  Bus Creator/1 -> Virtual/1
  Data Type Conversion/1 -> Bus Creator/1  "Voltage [V]"
  Data Type Conversion1/1 -> Bus Creator/2  "Current [mA]"
  Data Type Conversion2/1 -> Bus Creator/3  "Consumed Capacity [mAh]"
  Data Type Conversion3/1 -> Bus Creator/4  "Remaining Capacity [%]"
  Data Type Conversion4/1 -> Bus Creator/5  "Remaining Flight Time [s]"

== system quadplane_sim_conf/Flight Management Unit/Control Laws/Variant Subsystem/FMU Mini/Virtual to Non-Virtual Mapping4/Subsystem2 ==
  Non-Virtual : Inport  OutDataTypeStr=Bus: AnalogData
  Bus Creator : BusCreator  Inputs=1
  Bus Selector : BusSelector  OutputSignals=val
  Data Type Conversion : DataTypeConversion  OutDataTypeStr=double  SaturateOnIntegerOverflow=off  RndMeth=Floor
  Virtual : Outport
  wires:
  Non-Virtual/1 -> Bus Selector/1
  Bus Creator/1 -> Virtual/1
  Data Type Conversion/1 -> Bus Creator/1  "Values"
  Bus Selector/1 -> Data Type Conversion/1  "<val>"

== system quadplane_sim_conf/Flight Management Unit/Control Laws/Variant Subsystem/FMU Mini/Virtual to Non-Virtual Mapping4/Subsystem3 ==
  Non-Virtual : Inport  OutDataTypeStr=Bus: PwmCmd
  Bus Creator : BusCreator  Inputs=2
  Bus Selector : BusSelector  OutputSignals=cnt,cmd
  Data Type Conversion : DataTypeConversion  OutDataTypeStr=double  SaturateOnIntegerOverflow=off  RndMeth=Floor
  Data Type Conversion1 : DataTypeConversion  OutDataTypeStr=double  SaturateOnIntegerOverflow=off  RndMeth=Floor
  Virtual : Outport
  wires:
  Non-Virtual/1 -> Bus Selector/1
  Bus Selector/2 -> Data Type Conversion1/1  "<cmd>"
  Data Type Conversion1/1 -> Bus Creator/2  "Cmds"
  Data Type Conversion/1 -> Bus Creator/1  "Cnt"
  Bus Selector/1 -> Data Type Conversion/1  "<cnt>"
  Bus Creator/1 -> Virtual/1

== system quadplane_sim_conf/Flight Management Unit/Control Laws/Variant Subsystem/FMU Mini/Virtual to Non-Virtual Mapping4/Subsystem4 ==
  Non-Virtual : Inport  OutDataTypeStr=Bus: SbusCmd
  Bus Creator : BusCreator  Inputs=4
  Bus Selector : BusSelector  OutputSignals=cnt,cmd
  Data Type Conversion{,1..3} (4 alike) : DataTypeConversion  OutDataTypeStr=double  SaturateOnIntegerOverflow=off  RndMeth=Floor
  Ground : Ground
  Ground1 : Ground
  Virtual : Outport
  wires:
  Non-Virtual/1 -> Bus Selector/1
  Bus Creator/1 -> Virtual/1
  Bus Selector/1 -> Data Type Conversion2/1  "<cnt>"
  Bus Selector/2 -> Data Type Conversion3/1  "<cmd>"
  Data Type Conversion2/1 -> Bus Creator/3  "Cnt"
  Data Type Conversion3/1 -> Bus Creator/4  "Cmds"
  Data Type Conversion1/1 -> Bus Creator/2  "Ch 18"
  Data Type Conversion/1 -> Bus Creator/1  "Ch 17"
  Ground/1 -> Data Type Conversion/1
  Ground1/1 -> Data Type Conversion1/1

== system quadplane_sim_conf/Flight Management Unit/Control Laws/Variant Subsystem/FMU Mini/Virtual to Non-Virtual Mapping5/Virtual to Non-Virtual Mapping1 ==
  Virtual : Inport
  Bus Creator : BusCreator  Inputs=5  OutDataTypeStr=Bus: InceptorData
  Bus Selector : BusSelector  OutputSignals=New Data,Lost Frame,Failsafe,Channel Data
  Constant : Constant  OutDataTypeStr=boolean
  Data Type Conversion : DataTypeConversion  OutDataTypeStr=boolean  SaturateOnIntegerOverflow=off  RndMeth=Floor
  Data Type Conversion1 : DataTypeConversion  OutDataTypeStr=boolean  SaturateOnIntegerOverflow=off  RndMeth=Floor
  Data Type Conversion2 : DataTypeConversion  OutDataTypeStr=boolean  SaturateOnIntegerOverflow=off  RndMeth=Floor
  Data Type Conversion5 : DataTypeConversion  OutDataTypeStr=int16  SaturateOnIntegerOverflow=off  RndMeth=Floor
  Non-Virtual : Outport  OutDataTypeStr=Bus: InceptorData
  wires:
  Virtual/1 -> Bus Selector/1
  Bus Creator/1 -> Non-Virtual/1
  Bus Selector/1 -> Data Type Conversion/1  "<New Data>"
  Bus Selector/2 -> Data Type Conversion1/1  "<Lost Frame>"
  Bus Selector/3 -> Data Type Conversion2/1  "<Failsafe>"
  Bus Selector/4 -> Data Type Conversion5/1  "<Channel Data>"
  Constant/1 -> Bus Creator/1  "healthy"
  Data Type Conversion/1 -> Bus Creator/2  "new_data"
  Data Type Conversion1/1 -> Bus Creator/3  "lost_frame"
  Data Type Conversion2/1 -> Bus Creator/4  "failsafe"
  Data Type Conversion5/1 -> Bus Creator/5  "ch"

== system quadplane_sim_conf/Flight Management Unit/Control Laws/Variant Subsystem/FMU Mini/Virtual to Non-Virtual Mapping5/Virtual to Non-Virtual Mapping2 ==
  Virtual : Inport
  Bus Creator : BusCreator  Inputs=6
  Bus Selector : BusSelector  OutputSignals=New IMU Data,IMU Healthy,Die Temperature [C],Accelerometer [m/s/s],Gyro [rad/s]
  Constant : Constant  OutDataTypeStr=boolean
  Data Type Conversion : DataTypeConversion  OutDataTypeStr=boolean  SaturateOnIntegerOverflow=off  RndMeth=Floor
  Data Type Conversion1 : DataTypeConversion  OutDataTypeStr=boolean  SaturateOnIntegerOverflow=off  RndMeth=Floor
  Data Type Conversion4 : DataTypeConversion  OutDataTypeStr=single  SaturateOnIntegerOverflow=off  RndMeth=Floor
  Data Type Conversion5 : DataTypeConversion  OutDataTypeStr=single  SaturateOnIntegerOverflow=off  RndMeth=Floor
  Data Type Conversion7 : DataTypeConversion  OutDataTypeStr=single  SaturateOnIntegerOverflow=off  RndMeth=Floor
  Non-Virtual : Outport  OutDataTypeStr=Bus: ImuData
  wires:
  Bus Creator/1 -> Non-Virtual/1
  Virtual/1 -> Bus Selector/1
  Constant/1 -> Bus Creator/1  "installed"
  Data Type Conversion1/1 -> Bus Creator/2  "healthy"
  Data Type Conversion4/1 -> Bus Creator/4  "die_temp_c"
  Data Type Conversion7/1 -> Bus Creator/6  "gyro_radps"
  Data Type Conversion/1 -> Bus Creator/3  "new_data"
  Bus Selector/1 -> Data Type Conversion1/1  "<New IMU Data>"
  Bus Selector/2 -> Data Type Conversion/1  "<IMU Healthy>"
  Bus Selector/3 -> Data Type Conversion4/1  "<Die Temperature [C]>"
  Bus Selector/4 -> Data Type Conversion5/1  "<Accelerometer [m/s/s]>"
  Data Type Conversion5/1 -> Bus Creator/5  "accel_mps2"
  Bus Selector/5 -> Data Type Conversion7/1  "<Gyro [rad/s]>"

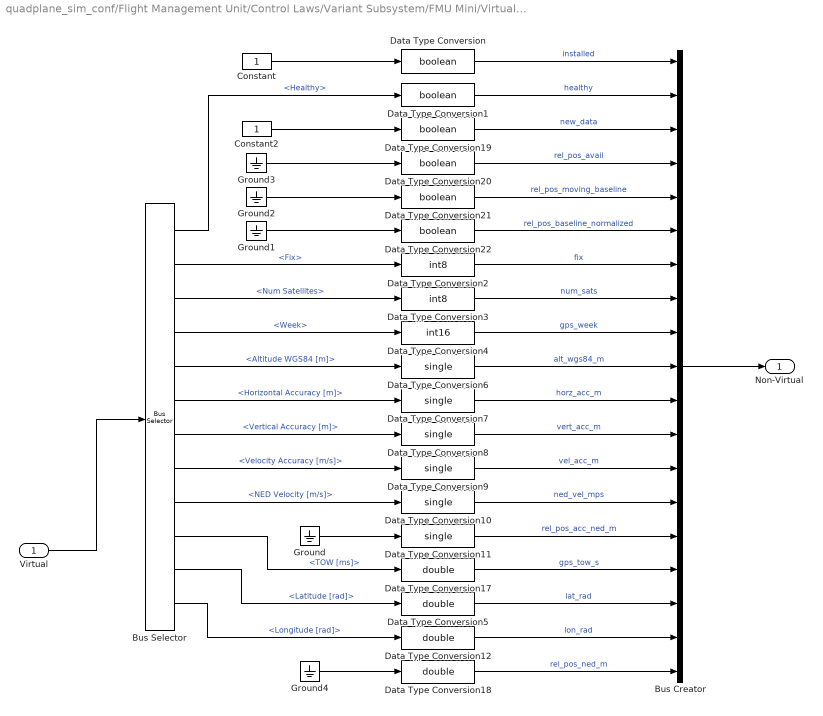
== system quadplane_sim_conf/Flight Management Unit/Control Laws/Variant Subsystem/FMU Mini/Virtual to Non-Virtual Mapping5/Virtual to Non-Virtual Mapping3 ==
  Virtual : Inport
  Bus Creator : BusCreator  Inputs=19  OutDataTypeStr=Bus: GnssData
  Bus Selector : BusSelector  OutputSignals=Healthy,Fix,Num Satellites,Week,Altitude WGS84 [m],Horizontal Accuracy [m],Vertical Accuracy [m],Velocity Accuracy [m/s],NED Velocity [m/s],TOW [ms],Latitude [rad],Longitude [rad]
  Constant : Constant  OutDataTypeStr=boolean
  Constant2 : Constant  OutDataTypeStr=boolean
  Data Type Conversion{,1,19..22} (6 alike) : DataTypeConversion  OutDataTypeStr=boolean  SaturateOnIntegerOverflow=off  RndMeth=Floor
  Data Type Conversion{6..11} (6 alike) : DataTypeConversion  OutDataTypeStr=single  SaturateOnIntegerOverflow=off  RndMeth=Floor
  Data Type Conversion{5,12,17..18} (4 alike) : DataTypeConversion  OutDataTypeStr=double  SaturateOnIntegerOverflow=off  RndMeth=Floor
  Data Type Conversion2 : DataTypeConversion  OutDataTypeStr=int8  SaturateOnIntegerOverflow=off  RndMeth=Floor
  Data Type Conversion3 : DataTypeConversion  OutDataTypeStr=int8  SaturateOnIntegerOverflow=off  RndMeth=Floor
  Data Type Conversion4 : DataTypeConversion  OutDataTypeStr=int16  SaturateOnIntegerOverflow=off  RndMeth=Floor
  Ground{,1..4} (5 alike) : Ground
  Non-Virtual : Outport  OutDataTypeStr=Bus: GnssData
  wires:
  Virtual/1 -> Bus Selector/1
  Bus Creator/1 -> Non-Virtual/1
  Data Type Conversion/1 -> Bus Creator/1  "installed"
  Data Type Conversion1/1 -> Bus Creator/2  "healthy"
  Data Type Conversion19/1 -> Bus Creator/3  "new_data"
  Data Type Conversion20/1 -> Bus Creator/4  "rel_pos_avail"
  Data Type Conversion21/1 -> Bus Creator/5  "rel_pos_moving_baseline"
  Data Type Conversion22/1 -> Bus Creator/6  "rel_pos_baseline_normalized"
  Data Type Conversion2/1 -> Bus Creator/7  "fix"
  Data Type Conversion3/1 -> Bus Creator/8  "num_sats"
  Data Type Conversion4/1 -> Bus Creator/9  "gps_week"
  Data Type Conversion6/1 -> Bus Creator/10  "alt_wgs84_m"
  Data Type Conversion7/1 -> Bus Creator/11  "horz_acc_m"
  Data Type Conversion8/1 -> Bus Creator/12  "vert_acc_m"
  Data Type Conversion9/1 -> Bus Creator/13  "vel_acc_m"
  Data Type Conversion10/1 -> Bus Creator/14  "ned_vel_mps"
  Data Type Conversion11/1 -> Bus Creator/15  "rel_pos_acc_ned_m"
  Data Type Conversion17/1 -> Bus Creator/16  "gps_tow_s"
  Data Type Conversion5/1 -> Bus Creator/17  "lat_rad"
  Data Type Conversion12/1 -> Bus Creator/18  "lon_rad"
  Data Type Conversion18/1 -> Bus Creator/19  "rel_pos_ned_m"
  Constant/1 -> Data Type Conversion/1
  Constant2/1 -> Data Type Conversion19/1
  Ground3/1 -> Data Type Conversion20/1
  Ground2/1 -> Data Type Conversion21/1
  Ground1/1 -> Data Type Conversion22/1
  Bus Selector/1 -> Data Type Conversion1/1  "<Healthy>"
  Bus Selector/2 -> Data Type Conversion2/1  "<Fix>"
  Bus Selector/3 -> Data Type Conversion3/1  "<Num Satellites>"
  Bus Selector/4 -> Data Type Conversion4/1  "<Week>"
  Bus Selector/5 -> Data Type Conversion6/1  "<Altitude WGS84 [m]>"
  Bus Selector/6 -> Data Type Conversion7/1  "<Horizontal Accuracy [m]>"
  Bus Selector/7 -> Data Type Conversion8/1  "<Vertical Accuracy [m]>"
  Bus Selector/8 -> Data Type Conversion9/1  "<Velocity Accuracy [m/s]>"
  Bus Selector/10 -> Data Type Conversion17/1  "<TOW [ms]>"
  Bus Selector/9 -> Data Type Conversion10/1  "<NED Velocity [m/s]>"
  Ground/1 -> Data Type Conversion11/1
  Bus Selector/11 -> Data Type Conversion5/1  "<Latitude [rad]>"
  Bus Selector/12 -> Data Type Conversion12/1  "<Longitude [rad]>"
  Ground4/1 -> Data Type Conversion18/1

== system quadplane_sim_conf/Flight Management Unit/Control Laws/Variant Subsystem/FMU Mini/Virtual to Non-Virtual Mapping5/Virtual to Non-Virtual Mapping4 ==
  Virtual : Inport
  Bus Creator : BusCreator  Inputs=6  OutDataTypeStr=Bus: PresData
  Bus Selector : BusSelector  OutputSignals=Healthy,New Data,Die Temperature [C],Pressure [Pa]
  Constant : Constant  OutDataTypeStr=boolean
  Constant1 : Constant  OutDataTypeStr=boolean
  Data Type Conversion : DataTypeConversion  OutDataTypeStr=boolean  SaturateOnIntegerOverflow=off  RndMeth=Floor
  Data Type Conversion1 : DataTypeConversion  OutDataTypeStr=boolean  SaturateOnIntegerOverflow=off  RndMeth=Floor
  Data Type Conversion2 : DataTypeConversion  OutDataTypeStr=single  SaturateOnIntegerOverflow=off  RndMeth=Floor
  Data Type Conversion3 : DataTypeConversion  OutDataTypeStr=single  SaturateOnIntegerOverflow=off  RndMeth=Floor
  Non-Virtual : Outport  OutDataTypeStr=Bus: PresData
  wires:
  Bus Creator/1 -> Non-Virtual/1
  Virtual/1 -> Bus Selector/1
  Bus Selector/2 -> Data Type Conversion/1  "<New Data>"
  Bus Selector/1 -> Data Type Conversion1/1  "<Healthy>"
  Bus Selector/4 -> Data Type Conversion2/1  "<Pressure [Pa]>"
  Bus Selector/3 -> Data Type Conversion3/1  "<Die Temperature [C]>"
  Constant/1 -> Bus Creator/1  "installed"
  Constant1/1 -> Bus Creator/2  "is_static_pres"
  Data Type Conversion1/1 -> Bus Creator/3  "healthy"
  Data Type Conversion/1 -> Bus Creator/4  "new_data"
  Data Type Conversion3/1 -> Bus Creator/5  "die_temp_c"
  Data Type Conversion2/1 -> Bus Creator/6  "pres_pa"

== system quadplane_sim_conf/Flight Management Unit/Control Laws/Variant Subsystem/FMU Mini/Virtual to Non-Virtual Mapping5/Virtual to Non-Virtual Mapping5 ==
  Virtual : Inport
  Bus Creator : BusCreator  Inputs=5  OutDataTypeStr=Bus: MagData
  Bus Selector : BusSelector  OutputSignals=Magnetometer Healthy,New Magnetometer Data,Die Temperature [C],Magnetometer [uT]
  Constant : Constant  OutDataTypeStr=boolean
  Data Type Conversion : DataTypeConversion  OutDataTypeStr=boolean  SaturateOnIntegerOverflow=off  RndMeth=Floor
  Data Type Conversion1 : DataTypeConversion  OutDataTypeStr=boolean  SaturateOnIntegerOverflow=off  RndMeth=Floor
  Data Type Conversion4 : DataTypeConversion  OutDataTypeStr=single  SaturateOnIntegerOverflow=off  RndMeth=Floor
  Data Type Conversion6 : DataTypeConversion  OutDataTypeStr=single  SaturateOnIntegerOverflow=off  RndMeth=Floor
  Non-Virtual : Outport  OutDataTypeStr=Bus: MagData
  wires:
  Virtual/1 -> Bus Selector/1
  Bus Creator/1 -> Non-Virtual/1
  Constant/1 -> Bus Creator/1  "installed"
  Data Type Conversion/1 -> Bus Creator/2  "healthy"
  Data Type Conversion1/1 -> Bus Creator/3  "new_data"
  Data Type Conversion4/1 -> Bus Creator/4  "die_temp_c"
  Data Type Conversion6/1 -> Bus Creator/5  "mag_ut"
  Bus Selector/1 -> Data Type Conversion/1  "<Magnetometer Healthy>"
  Bus Selector/2 -> Data Type Conversion1/1  "<New Magnetometer Data>"
  Bus Selector/3 -> Data Type Conversion4/1  "<Die Temperature [C]>"
  Bus Selector/4 -> Data Type Conversion6/1  "<Magnetometer [uT]>"

== system quadplane_sim_conf/Flight Management Unit/Control Laws/Variant Subsystem/FMU Mini/Virtual to Non-Virtual Mapping5/Virtual to Non-Virtual Mapping6 ==
  Virtual : Inport
  Bus Creator : BusCreator  Inputs=1
  Bus Selector : BusSelector  OutputSignals=Voltages
  Data Type Conversion2 : DataTypeConversion  OutDataTypeStr=single  SaturateOnIntegerOverflow=off  RndMeth=Floor
  Non-Virtual : Outport  OutDataTypeStr=Bus: AdcData
  wires:
  Bus Creator/1 -> Non-Virtual/1
  Virtual/1 -> Bus Selector/1
  Data Type Conversion2/1 -> Bus Creator/1  "volt"
  Bus Selector/1 -> Data Type Conversion2/1  "<Voltages>"

== system quadplane_sim_conf/Flight Management Unit/Control Laws/Variant Subsystem/FMU Mini/Virtual to Non-Virtual Mapping5/Virtual to Non-Virtual Mapping7 ==
  Virtual : Inport
  Bus Creator : BusCreator  Inputs=2
  Bus Selector : BusSelector  OutputSignals=Voltage [V],Current [V]
  Data Type Conversion1 : DataTypeConversion  OutDataTypeStr=single  SaturateOnIntegerOverflow=off  RndMeth=Floor
  Data Type Conversion2 : DataTypeConversion  OutDataTypeStr=single  SaturateOnIntegerOverflow=off  RndMeth=Floor
  Non-Virtual : Outport  OutDataTypeStr=Bus: PowerModuleData
  wires:
  Virtual/1 -> Bus Selector/1
  Bus Creator/1 -> Non-Virtual/1
  Bus Selector/1 -> Data Type Conversion1/1  "<Voltage [V]>"
  Data Type Conversion1/1 -> Bus Creator/1  "voltage_v"
  Bus Selector/2 -> Data Type Conversion2/1  "<Current [V]>"
  Data Type Conversion2/1 -> Bus Creator/2  "current_ma"
